simulink model "untitled"  (R2022b)
settings: Solver=FixedStepDiscrete  StartTime=0.0  StopTime=10.0  RelTol=1e-3
undefined symbols (not defined in the file): D1, P
settings Model: Creator=EDKI  LastModifiedBy=EDKI

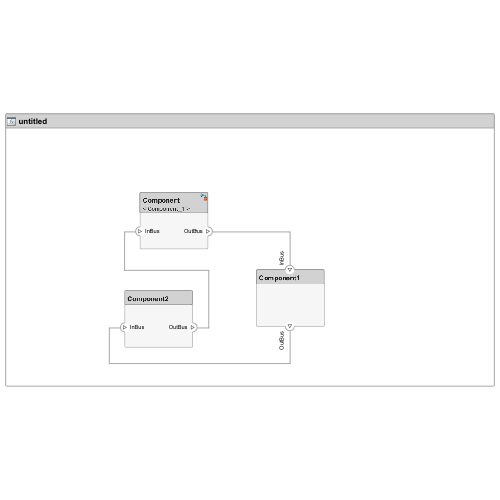
[thumbnail: Simulink's stored preview of the top-level diagram]
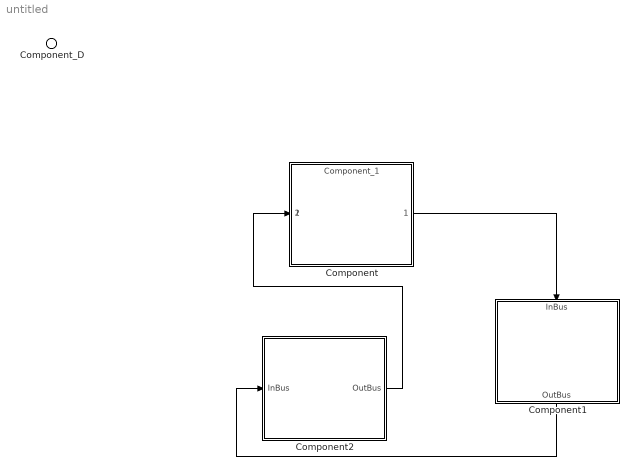
== system untitled ==
  Component_D : Inport  OutputFunctionCall=on
  Component : ModelReference  ModelNameDialog=Component_1  SimulationMode=Normal  ScheduleRates=on  ModelEventPortInfo=P:D1[-2][0][0]  ModelReferenceVersion=1.2
      settings: PortSchema="{\"entries\":[{\"content\":{\"headerSize\":38,\"margin\":15,\"minimumSpacing\":25,\"sides\":[{\"content\":{\"connectorIds\":[\"In1\"]},\"type\":\"ConnectorPlacement.EquallySpacedRectSide\",\"uuid\":\"30c282d5-1b70-4352-aa58-9b273f67781a\"},{\"content\":{\"connectorIds\":[\"Out1\"],\"side\":\"RIGHT\"},\"type\":\"ConnectorPlacement.EquallySpacedRectSide\",\"uuid\":\"86ff41a1-9909-4d6d-8af3-93663d3dc2ec\"},{\"content\":{\"connectorIds\":[],\"side\":\"TOP\"},\"type\":\"ConnectorPlacement.EquallySpacedRectSide\",\"uuid\":\"8cda0cbc-90f4-4c0e-b448-b417a24de224\"},{\"content\":{\"connectorIds\":[\"In2\"],\"side\":\"HIDDEN\"},\"type\":\"ConnectorPlacement.EquallySpacedRectSide\",\"uuid\":\"f4e101d5-6d34-49dc-ab2f-923c8885429b\"}]},\"type\":\"ConnectorPlacement.EquallySpacedConnector\",\"uuid\":\"9c681b32-5981-44d2-8851-b301e75603c9\"}],\"packageUris\":[\"http://schema.mathworks.com/mf0/Connector/R2020b\"],\"version\":\"1.0\"}"
  Component1 : Subsystem
      settings: PortSchema="{\"entries\":[{\"content\":{\"headerSize\":26,\"margin\":15,\"minimumSpacing\":25,\"sides\":[{\"content\":{\"connectorIds\":[]},\"type\":\"ConnectorPlacement.EquallySpacedRectSide\",\"uuid\":\"30c282d5-1b70-4352-aa58-9b273f67781a\"},{\"content\":{\"connectorIds\":[],\"side\":\"RIGHT\"},\"type\":\"ConnectorPlacement.EquallySpacedRectSide\",\"uuid\":\"86ff41a1-9909-4d6d-8af3-93663d3dc2ec\"},{\"content\":{\"connectorIds\":[\"In1\"],\"side\":\"TOP\"},\"type\":\"ConnectorPlacement.EquallySpacedRectSide\",\"uuid\":\"8cda0cbc-90f4-4c0e-b448-b417a24de224\"},{\"content\":{\"connectorIds\":[\"Out1\"],\"side\":\"BOTTOM\"},\"type\":\"ConnectorPlacement.EquallySpacedRectSide\",\"uuid\":\"9aa25b61-5916-4557-b229-8c17e47d3bf5\"}]},\"type\":\"ConnectorPlacement.EquallySpacedConnector\",\"uuid\":\"9c681b32-5981-44d2-8851-b301e75603c9\"}],\"packageUris\":[\"http://schema.mathworks.com/mf0/Connector/R2020b\"],\"version\":\"1.0\"}"
  Component2 : Subsystem
      settings: PortSchema="{\"entries\":[{\"content\":{\"headerSize\":26,\"margin\":15,\"minimumSpacing\":25,\"sides\":[{\"content\":{\"connectorIds\":[\"In1\"]},\"type\":\"ConnectorPlacement.EquallySpacedRectSide\",\"uuid\":\"30c282d5-1b70-4352-aa58-9b273f67781a\"},{\"content\":{\"connectorIds\":[\"Out1\"],\"side\":\"RIGHT\"},\"type\":\"ConnectorPlacement.EquallySpacedRectSide\",\"uuid\":\"86ff41a1-9909-4d6d-8af3-93663d3dc2ec\"},{\"content\":{\"connectorIds\":[],\"side\":\"TOP\"},\"type\":\"ConnectorPlacement.EquallySpacedRectSide\",\"uuid\":\"8cda0cbc-90f4-4c0e-b448-b417a24de224\"}]},\"type\":\"ConnectorPlacement.EquallySpacedConnector\",\"uuid\":\"9c681b32-5981-44d2-8851-b301e75603c9\"}],\"packageUris\":[\"http://schema.mathworks.com/mf0/Connector/R2020b\"],\"version\":\"1.0\"}"
  wires:
  Component1/1(OutBus) -> Component2/1(InBus)
  Component2/1(OutBus) -> Component/1
  Component/1 -> Component1/1(InBus)

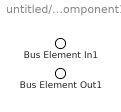
== system untitled/Component1 ==
  Bus Element In1 : Inport  PortName=InBus
  Bus Element Out1 : Outport  PortName=OutBus

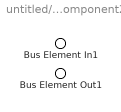
== system untitled/Component2 ==
  Bus Element In1 : Inport  PortName=InBus
  Bus Element Out1 : Outport  PortName=OutBus
